simulink model "cpp_m1hp_demo"  (R2022b)
settings: Solver=FixedStepDiscrete  StartTime=0.0  StopTime=6  FixedStep=FEM_Ts  MaxStep=FEM_Ts  RelTol=1e-2
InitFcn:
  | %
  | % Initialization callback function
  | %
  | 
  | try
  |    fprintf('\nGMT IMS version (%s)!\n',simulink_fname );
  | 
  |    % Get Simulink model directory
  |    [filepath,name,ext] = fileparts(which(bdroot));
  | 
  |    if ~strcmp(filepath,pwd)
  |       fprintf('\nChanging current directory to \n %s \n',filepath);
  |       cd(filepath);
  |    end
  | 
  |    %
  |  if(osim.bpless_wl)
  |     fprintf('Generating bumpless wind load time series\n');
  |  end
  | catch
  |    warning('Running the InitFcn from puSimulate script');
  | end
values from neighbouring files (symbols this model uses):
  a_max = 250e-6    (= 0.00025)    [load_im_with_m1act_damp.m]    (also in load_m1hp_cpp_demo.m)
  b = B(:,in)*m1sys{seg}.Kbal    [evalM1ofl_act_damp.m]
  c = [Upsilon*C(out0,:);     C(out1a,:)-C(out1b,:);     C(out2,:)]    [evalM1ofl_act_damp.m]
  delta_sim = 1e-3    (= 0.001)    [load_im_with_m1act_damp.m]    (also in load_m1hp_cpp_demo.m)
  drv_delay = ceil(mount.delay/FEM_Ts)    [load_im_with_m1act_damp.m]    (also in load_m1hp_cpp_demo.m)
  FEM_Ts = 1/1e3    (= 0.001)    [load_im_with_m1act_damp.m]    (also in load_m1hp_cpp_demo.m)
  Hdrive_d = c2d(o.Hdrive(1,1), FEM_Ts, 'tustin')    [load_im_with_m1act_damp.m]    (also in load_m1hp_cpp_demo.m)
  m1sys = ovr_ofl_crtl(m1sys,seg)    [evalM1ofl_act_damp.m]    (also in load_im_with_m1act_damp.m = ovr_ofl_crtl(m1sys))
  o = fun_confBase(oTest)    [load_im_with_m1act_damp.m]    (also in load_m1hp_cpp_demo.m)
  PG = zeros(length(om2),6)    [load_im_with_m1act_damp.m]    (also in load_m1hp_cpp_demo.m)
  phiB = inputs2ModalF(mode_ind_vec,indDesInputs)    [load_im_with_m1act_damp.m]    (also in load_m1hp_cpp_demo.m)
  phiC = modalDisp2Outputs(indDesOutputs,mode_ind_vec)    [load_im_with_m1act_damp.m]    (also in load_m1hp_cpp_demo.m)
  Psi_ss = gainMatrix(indDesOutputs,indDesInputs) - K_ss    [load_im_with_m1act_damp.m]    (also in load_m1hp_cpp_demo.m)
  t_gd = 0*0.5    (= 0)    [load_im_with_m1act_damp.m]    (also in load_m1hp_cpp_demo.m)
  t_gd_v = 0*t_gd    (= 0)    [load_im_with_m1act_damp.m]    (also in load_m1hp_cpp_demo.m)
  Tcmd = 12    [load_im_with_m1act_damp.m]    (also in load_m1hp_cpp_demo.m)
  v0 = 0    [load_im_with_m1act_damp.m]    (also in load_m1hp_cpp_demo.m)
  v_max = 50e-6    (= 5e-05)    [load_im_with_m1act_damp.m]    (also in load_m1hp_cpp_demo.m)
  x0 = 0    [load_im_with_m1act_damp.m]    (also in load_m1hp_cpp_demo.m)
  x0_f = xf(end,:)    [load_im_with_m1act_damp.m]    (also in load_m1hp_cpp_demo.m)
undefined symbols (not defined in the file or in its folder): a, A_f, az, az_ff_en, B_f, C_f, D_f, DiscIntNeverNeededParam, el, gir, magnitude, mount, osim
libraries: simulink x8, ims_block_library x7, simulink_extras x2
(part 1 of 3)
settings Model: PauseTimes=0  Creator=RRomano  LastModifiedBy=rromano
settings SolverCC: MaxConsecutiveMinStep=10  ZeroCrossAlgorithm=Adaptive  AlgebraicLoopSolver=TrustRegion
settings DataIOCC: SaveOutput=off  SignalLogging=off  DSMLogging=off  SaveTime=off  ReturnWorkspaceOutputs=off
settings OptimizationCC: DefaultParameterBehavior=Inlined  StrengthReduction=on  PassReuseOutputArgsAs=Individual arguments  EfficientMapNaN2IntZero=off  SimCompilerOptimization=on  AccelVerboseBuild=on  OptimizeBlockOrder=speed  OptimizationPriority=Speed  OptimizationCustomize=off  MultiThreadedLoops=on  EfficientTunableParamExpr=on
settings DebuggingCC: InheritedTsInSrcMsg=none  MultiTaskRateTransMsg=warning  ParameterTunabilityLossMsg=error  UnconnectedInputMsg=warning  UnconnectedOutputMsg=warning  UnconnectedLineMsg=warning  SFUnexpectedBacktrackingDiag=warning  SFNoUnconditionalDefaultTransitionDiag=warning  SFExecutionAtInitializationDiag=none  SFMachineParentedDataDiag=warning  ArithmeticOperatorsInVariantConditions=warning
settings HardwareCC: ProdBitPerLong=64  ProdHWDeviceType=Intel->x86-64 (Linux 64)  TargetBitPerLong=64  TargetBitPerPointer=64  TargetBitPerSizeT=64  TargetBitPerPtrDiffT=64  TargetLongLongMode=on  TargetIntDivRoundTo=Zero  TargetEndianess=LittleEndian  TargetWordSize=64  TargetHWDeviceType=MATLAB Host  ProdEqTarget=off
settings ModelReferenceCC: EnableRefExpFcnMdlSchedulingChecks=on
settings SFSimCC: SimUseLocalCustomCode=off  MATLABDynamicMemAlloc=off  CustomCodeUndefinedFunction=UseInterfaceOnly
settings RTWCC: Description=Embedded Coder  SystemTargetFile=ert.tlc  GenCodeOnly=on  TemplateMakefile=ert_default_tmf  GenerateReport=on  BuildConfiguration=Faster Runs  IncludeHyperlinkInReport=on  GenerateTraceInfo=on  GenerateTraceReport=on  GenerateTraceReportSl=on  GenerateTraceReportSf=on  GenerateTraceReportEml=on  DLArmComputeVersion=19.05
settings CodeAppCC: ForceParamTrailComments=on  IgnoreCustomStorageClasses=off  MaxIdLength=128  OperatorAnnotations=on  SimulinkDataObjDesc=on  SFDataObjDesc=on  InsertBlockDesc=on  MATLABSourceComments=on
settings ERTTargetCC: GenerateSampleERTMain=on  InlinedParameterPlacement=NonHierarchical  ERTCustomFileTemplate=example_file_process.tlc
settings ConfigComp: CovMetricSettings=dw  CovSaveCumulativeToWorkspaceVar=on  CovSaveSingleToWorkspaceVar=on  CovExternalEMLEnable=off

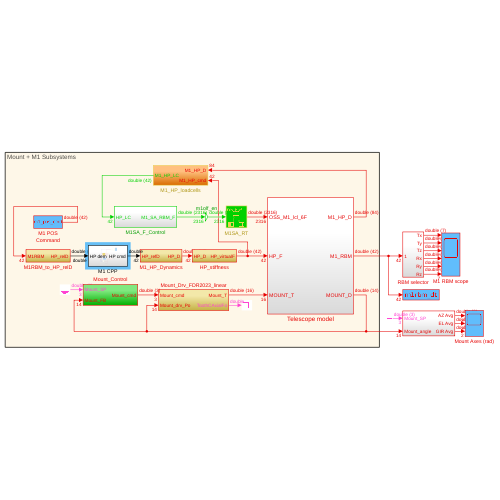
[thumbnail: Simulink's stored preview of the top-level diagram]
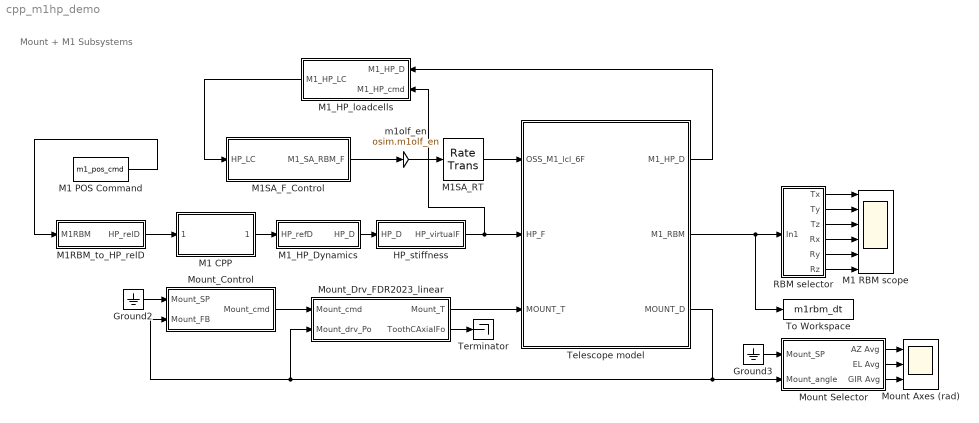
== system cpp_m1hp_demo ==
  note: Mount + M1 Subsystems
  Ground2 : Ground
  Ground3 : Ground
  HP_stiffness : Subsystem
  M1 CPP : Subsystem
  M1 POS Command : FromWorkspace  VariableName=m1_pos_cmd  SampleTime=-1  Interpolate=off  OutputAfterFinalValue=Holding final value
  M1 RBM scope : Scope  NumInputPorts=6
  M1RBM_to_HP_relD : Subsystem
  M1SA_F_Control : Subsystem
  M1SA_RT : RateTransition  Deterministic=off  OutPortSampleTime=FEM_Ts
  M1_HP_Dynamics : Subsystem
  M1_HP_loadcells : Subsystem
  Mount Axes (rad) : Scope  NumInputPorts=3
  Mount Selector : Subsystem
  Mount_Control : Subsystem
  Mount_Drv_FDR2023_linear : Subsystem
  RBM selector : Subsystem
  Telescope model : Subsystem
  Terminator : Terminator
  To Workspace : ToWorkspace  VariableName=m1rbm_dt  SampleTime=-1
  m1olf_en : Gain  Gain=osim.m1olf_en
  wires:
  M1_HP_Dynamics/1(HP_D) -> HP_stiffness/1(HP_D)
  M1SA_F_Control/1(M1_SA_RBM_F) -> m1olf_en/1
  Ground2/1 -> Mount_Control/1(Mount_SP)
  M1_HP_loadcells/1(M1_HP_LC) -> M1SA_F_Control/1(HP_LC)
  Telescope model/3(MOUNT_D) -> Mount Selector/2(Mount_angle), Mount_Drv_FDR2023_linear/2(Mount_drv_Po), Mount_Control/2(Mount_FB)
  Mount_Drv_FDR2023_linear/2(ToothCAxialFo) -> Terminator/1
  Telescope model/1(M1_HP_D) -> M1_HP_loadcells/1(M1_HP_D)
  Mount_Control/1(Mount_cmd) -> Mount_Drv_FDR2023_linear/1(Mount_cmd)
  Mount_Drv_FDR2023_linear/1(Mount_T) -> Telescope model/3(MOUNT_T)
  HP_stiffness/1(HP_virtualF) -> M1_HP_loadcells/2(M1_HP_cmd), Telescope model/2(HP_F)
  RBM selector/1(Tx) -> M1 RBM scope/1
  RBM selector/2(Ty) -> M1 RBM scope/2
  RBM selector/3(Tz) -> M1 RBM scope/3
  RBM selector/4(Rx) -> M1 RBM scope/4
  RBM selector/5(Ry) -> M1 RBM scope/5
  RBM selector/6(Rz) -> M1 RBM scope/6
  Telescope model/2(M1_RBM) -> To Workspace/1, RBM selector/1(In1)
  M1 POS Command/1 -> M1RBM_to_HP_relD/1(M1RBM)
  Mount Selector/1(AZ Avg) -> Mount Axes (rad)/1
  Mount Selector/2(EL Avg) -> Mount Axes (rad)/2
  Mount Selector/3(GIR Avg) -> Mount Axes (rad)/3
  Ground3/1 -> Mount Selector/1(Mount_SP)
  M1SA_RT/1 -> Telescope model/1(OSS_M1_lcl_6F)
  m1olf_en/1 -> M1SA_RT/1
  M1RBM_to_HP_relD/1(HP_relD) -> M1 CPP/1(HP dem)
  M1 CPP/1(HP cmd) -> M1_HP_Dynamics/1(HP_refD)

== system cpp_m1hp_demo/HP_stiffness ==
  note: This block takes HP reference relative displacements (lengths) and provides the virtual forces to enforce such a displacement. The force output also corrects (offsets) the HP load cell measurement by the commanded change in position.
  note: Offset displacement, used in calculation of hard point forces.
  note: The virtual force simulates the extension
      | of the HP by applying and equal and
      | opposite force on the face of the mirror and cell.
  note: HP virtual
      | forces (N)
  HP_D : Inport
  Demux1 : Demux  Outputs=6*ones(7,1)
  HpK1 : Gain  Gain=m1sys{2}.HPstiff
  HpK2 : Gain  Gain=m1sys{3}.HPstiff
  HpK3 : Gain  Gain=m1sys{5}.HPstiff
  HpK4 : Gain  Gain=m1sys{6}.HPstiff
  HpK5 : Gain  Gain=m1sys{4}.HPstiff
  HpK6 : Gain  Gain=m1sys{7}.HPstiff
  HpK8 : Gain  Gain=m1sys{1}.HPstiff
  Mux3 : Mux  Inputs=6*ones(7,1)
  HP_virtualF : Outport  VectorParamsAs1DForOutWhenUnconnected=off
  wires:
  Mux3/1 -> HP_virtualF/1
  HpK8/1 -> Mux3/1
  HpK6/1 -> Mux3/7
  HpK1/1 -> Mux3/2
  HpK2/1 -> Mux3/3
  HpK5/1 -> Mux3/4
  HpK3/1 -> Mux3/5
  HpK4/1 -> Mux3/6
  Demux1/1 -> HpK8/1
  HP_D/1 -> Demux1/1
  Demux1/2 -> HpK1/1
  Demux1/3 -> HpK2/1
  Demux1/4 -> HpK5/1
  Demux1/5 -> HpK3/1
  Demux1/6 -> HpK4/1
  Demux1/7 -> HpK6/1

== system cpp_m1hp_demo/M1 CPP ==
  HP dem : Inport
  Constant : Constant  Value=osim.m1cpp_en  VectorParams1D=off
  Ground1 : Ground
  HP scope : Scope  NumInputPorts=6
  HP selector : Subsystem
  M1CPP_RT : RateTransition  Integrity=off  Deterministic=off  OutPortSampleTime=Tcmd
  M1CPP_RT1 : RateTransition  Integrity=off  Deterministic=off
  Mux2 : Mux  Inputs=2
  Mux3 : Mux  Inputs=2
  Selector : Selector  InputPortWidth=42  IndexOptions=Index vector (dialog)  Indices=[7:42]  OutputSizes=1
  Selector1 : Selector  InputPortWidth=42  IndexOptions=Index vector (dialog)  Indices=[1:6]  OutputSizes=1
  Switch : Switch  Criteria=u2 ~= 0  SaturateOnIntegerOverflow=off  InputSameDT=off
  Terminator1 : Terminator
  Terminator2 : Terminator
  cmd_pre_proc : Subsystem
  HP cmd : Outport
  wires:
  HP selector/3(HP3) -> HP scope/3
  HP selector/2(HP2) -> HP scope/2
  HP selector/1(HP1) -> HP scope/1
  cmd_pre_proc/2(vel_d) -> Terminator1/1
  Switch/1 -> HP cmd/1
  HP selector/5(HP5) -> HP scope/5
  Mux3/1 -> M1CPP_RT1/1
  HP selector/6(HP6) -> HP scope/6
  HP selector/4(HP4) -> HP scope/4
  HP dem/1 -> Switch/3, M1CPP_RT/1
  cmd_pre_proc/3(acc_d) -> Terminator2/1
  M1CPP_RT1/1 -> Switch/1
  Selector/1 -> Mux3/2
  Selector1/1 -> cmd_pre_proc/1(x_target), Mux2/1
  Ground1/1 -> cmd_pre_proc/2(v_target)
  Constant/1 -> Switch/2
  M1CPP_RT/1 -> Selector/1, Selector1/1
  Mux2/1 -> HP selector/1(In1)
  cmd_pre_proc/1(pos_d) -> Mux2/2, Mux3/1

== system cpp_m1hp_demo/M1RBM_to_HP_relD ==
  note: CG desired
      | displacement/rotation
  note: This block converts from CG displacements and rotations,
      | and converts to Hard Point lengths.  Hard point lengths are
      | changed by applying an equal and opposite force to the hard
      | point, and then offseting output by the commanded change
      | in position.
  note: Hexapod Desired
      | Displacements
  note: Offset displacement, used in calculation of hard point forces.
  M1RBM : Inport
  CG2HpS1 : Gain  Gain=m1sys{1}.M1RBM2HP  Multiplication=Matrix(K*u)
  CG2HpS2 : Gain  Gain=m1sys{2}.M1RBM2HP  Multiplication=Matrix(K*u)
  CG2HpS3 : Gain  Gain=m1sys{3}.M1RBM2HP  Multiplication=Matrix(K*u)
  CG2HpS4 : Gain  Gain=m1sys{4}.M1RBM2HP  Multiplication=Matrix(K*u)
  CG2HpS5 : Gain  Gain=m1sys{5}.M1RBM2HP  Multiplication=Matrix(K*u)
  CG2HpS6 : Gain  Gain=m1sys{6}.M1RBM2HP  Multiplication=Matrix(K*u)
  CG2HpS7 : Gain  Gain=m1sys{7}.M1RBM2HP  Multiplication=Matrix(K*u)
  Demux1 : Demux  Outputs=6*ones(7,1)
  Mux3 : Mux  Inputs=6*ones(7,1)
  HP_relD : Outport  VectorParamsAs1DForOutWhenUnconnected=off
  wires:
  Mux3/1 -> HP_relD/1
  Demux1/2 -> CG2HpS2/1
  Demux1/3 -> CG2HpS3/1
  Demux1/4 -> CG2HpS4/1
  Demux1/5 -> CG2HpS5/1
  Demux1/6 -> CG2HpS6/1
  Demux1/1 -> CG2HpS1/1
  Demux1/7 -> CG2HpS7/1
  CG2HpS1/1 -> Mux3/1
  M1RBM/1 -> Demux1/1
  CG2HpS2/1 -> Mux3/2
  CG2HpS3/1 -> Mux3/3
  CG2HpS4/1 -> Mux3/4
  CG2HpS5/1 -> Mux3/5
  CG2HpS6/1 -> Mux3/6
  CG2HpS7/1 -> Mux3/7

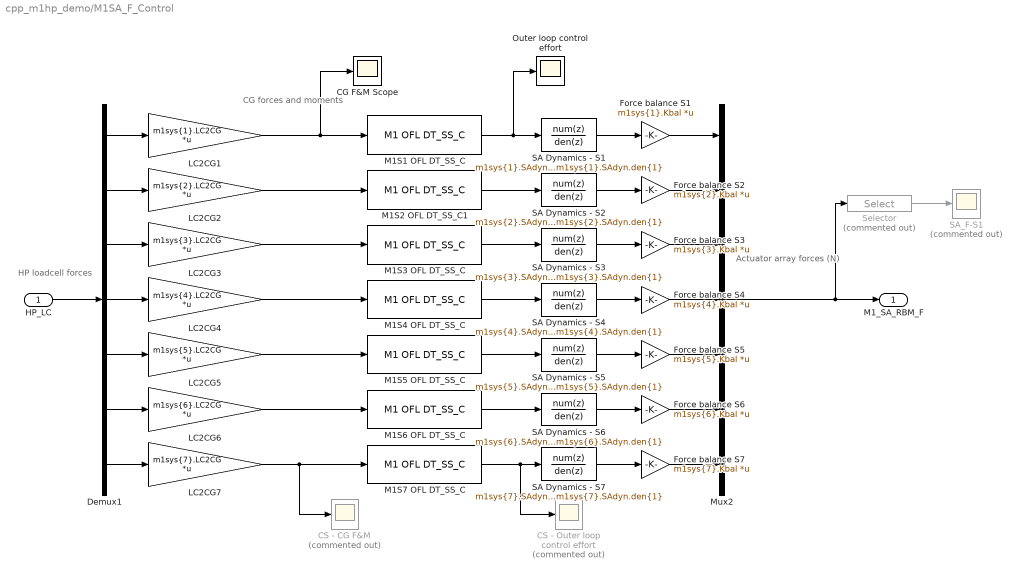
== system cpp_m1hp_demo/M1SA_F_Control ==
  note: HP loadcell forces
  note: Actuator array
      | forces (N)
  note: CG forces
      | and moments
  HP_LC : Inport
  CG F&M Scope : Scope
  CS - CG F&M : Scope  Commented=on
  CS - Outer loop control effort : Scope  Commented=on
  Demux1 : Demux  Outputs=6*ones(7,1)
  Force balance S1 : Gain  Gain=m1sys{1}.Kbal  Multiplication=Matrix(K*u)
  Force balance S2 : Gain  Gain=m1sys{2}.Kbal  Multiplication=Matrix(K*u)
  Force balance S3 : Gain  Gain=m1sys{3}.Kbal  Multiplication=Matrix(K*u)
  Force balance S4 : Gain  Gain=m1sys{4}.Kbal  Multiplication=Matrix(K*u)
  Force balance S5 : Gain  Gain=m1sys{5}.Kbal  Multiplication=Matrix(K*u)
  Force balance S6 : Gain  Gain=m1sys{6}.Kbal  Multiplication=Matrix(K*u)
  Force balance S7 : Gain  Gain=m1sys{7}.Kbal  Multiplication=Matrix(K*u)
  LC2CG1 : Gain  Gain=m1sys{1}.LC2CG  Multiplication=Matrix(K*u)
  LC2CG2 : Gain  Gain=m1sys{2}.LC2CG  Multiplication=Matrix(K*u)
  LC2CG3 : Gain  Gain=m1sys{3}.LC2CG  Multiplication=Matrix(K*u)
  LC2CG4 : Gain  Gain=m1sys{4}.LC2CG  Multiplication=Matrix(K*u)
  LC2CG5 : Gain  Gain=m1sys{5}.LC2CG  Multiplication=Matrix(K*u)
  LC2CG6 : Gain  Gain=m1sys{6}.LC2CG  Multiplication=Matrix(K*u)
  LC2CG7 : Gain  Gain=m1sys{7}.LC2CG  Multiplication=Matrix(K*u)
  M1S1 OFL DT_SS_C : ims_block_library/M1 OFL DT_SS_C  dt_SS_struct=m1sys{1}.ofl.SSdtC
  M1S2 OFL DT_SS_C1 : ims_block_library/M1 OFL DT_SS_C  dt_SS_struct=m1sys{2}.ofl.SSdtC
  M1S3 OFL DT_SS_C : ims_block_library/M1 OFL DT_SS_C  dt_SS_struct=m1sys{3}.ofl.SSdtC
  M1S4 OFL DT_SS_C : ims_block_library/M1 OFL DT_SS_C  dt_SS_struct=m1sys{4}.ofl.SSdtC
  M1S5 OFL DT_SS_C : ims_block_library/M1 OFL DT_SS_C  dt_SS_struct=m1sys{5}.ofl.SSdtC
  M1S6 OFL DT_SS_C : ims_block_library/M1 OFL DT_SS_C  dt_SS_struct=m1sys{6}.ofl.SSdtC
  M1S7 OFL DT_SS_C : ims_block_library/M1 OFL DT_SS_C  dt_SS_struct=m1sys{7}.ofl.SSdtC
  Mux2 : Mux  Inputs=7
  Outer loop control effort : Scope
  SA Dynamics - S1 : DiscreteTransferFcn  Numerator=m1sys{1}.SAdyn.num{1}  Denominator=m1sys{1}.SAdyn.den{1}  SampleTime=m1sys{1}.ofl.Ts  a0EqualsOne=on
  SA Dynamics - S2 : DiscreteTransferFcn  Numerator=m1sys{2}.SAdyn.num{1}  Denominator=m1sys{2}.SAdyn.den{1}  SampleTime=m1sys{1}.ofl.SSdtC{1}.Ts  a0EqualsOne=on
  SA Dynamics - S3 : DiscreteTransferFcn  Numerator=m1sys{3}.SAdyn.num{1}  Denominator=m1sys{3}.SAdyn.den{1}  SampleTime=m1sys{1}.ofl.SSdtC{1}.Ts  a0EqualsOne=on
  SA Dynamics - S4 : DiscreteTransferFcn  Numerator=m1sys{4}.SAdyn.num{1}  Denominator=m1sys{4}.SAdyn.den{1}  SampleTime=m1sys{1}.ofl.SSdtC{1}.Ts  a0EqualsOne=on
  SA Dynamics - S5 : DiscreteTransferFcn  Numerator=m1sys{5}.SAdyn.num{1}  Denominator=m1sys{5}.SAdyn.den{1}  SampleTime=m1sys{1}.ofl.SSdtC{1}.Ts  a0EqualsOne=on
  SA Dynamics - S6 : DiscreteTransferFcn  Numerator=m1sys{6}.SAdyn.num{1}  Denominator=m1sys{6}.SAdyn.den{1}  SampleTime=m1sys{1}.ofl.SSdtC{1}.Ts  a0EqualsOne=on
  SA Dynamics - S7 : DiscreteTransferFcn  Numerator=m1sys{7}.SAdyn.num{1}  Denominator=m1sys{7}.SAdyn.den{1}  SampleTime=m1sys{1}.ofl.SSdtC{1}.Ts  a0EqualsOne=on
  SA_F-S1 : Scope  Commented=on
  Selector : Selector  Commented=on  InputPortWidth=2316  IndexOptions=Index vector (dialog)  Indices=[1:335]  OutputSizes=1
  M1_SA_RBM_F : Outport  VectorParamsAs1DForOutWhenUnconnected=off
  wires:
  HP_LC/1 -> Demux1/1
  M1S1 OFL DT_SS_C/1 -> Outer loop control effort/1, SA Dynamics - S1/1
  M1S2 OFL DT_SS_C1/1 -> SA Dynamics - S2/1
  M1S3 OFL DT_SS_C/1 -> SA Dynamics - S3/1
  M1S4 OFL DT_SS_C/1 -> SA Dynamics - S4/1
  M1S5 OFL DT_SS_C/1 -> SA Dynamics - S5/1
  M1S6 OFL DT_SS_C/1 -> SA Dynamics - S6/1
  M1S7 OFL DT_SS_C/1 -> CS - Outer loop control effort/1, SA Dynamics - S7/1
  LC2CG7/1 -> M1S7 OFL DT_SS_C/1, CS - CG F&M/1
  LC2CG6/1 -> M1S6 OFL DT_SS_C/1
  LC2CG5/1 -> M1S5 OFL DT_SS_C/1
  LC2CG4/1 -> M1S4 OFL DT_SS_C/1
  LC2CG3/1 -> M1S3 OFL DT_SS_C/1
  LC2CG2/1 -> M1S2 OFL DT_SS_C1/1
  LC2CG1/1 -> M1S1 OFL DT_SS_C/1, CG F&M Scope/1
  Demux1/1 -> LC2CG1/1
  Demux1/2 -> LC2CG2/1
  Demux1/3 -> LC2CG3/1
  Demux1/4 -> LC2CG4/1
  Demux1/5 -> LC2CG5/1
  Demux1/6 -> LC2CG6/1
  Demux1/7 -> LC2CG7/1
  Force balance S2/1 -> Mux2/2
  Force balance S3/1 -> Mux2/3
  Force balance S4/1 -> Mux2/4
  Force balance S6/1 -> Mux2/6
  Force balance S5/1 -> Mux2/5
  Force balance S7/1 -> Mux2/7
  Mux2/1 -> M1_SA_RBM_F/1, Selector/1
  SA Dynamics - S1/1 -> Force balance S1/1
  SA Dynamics - S2/1 -> Force balance S2/1
  SA Dynamics - S3/1 -> Force balance S3/1
  SA Dynamics - S4/1 -> Force balance S4/1
  SA Dynamics - S5/1 -> Force balance S5/1
  SA Dynamics - S6/1 -> Force balance S6/1
  SA Dynamics - S7/1 -> Force balance S7/1
  Selector/1 -> SA_F-S1/1
  Force balance S1/1 -> Mux2/1

== system cpp_m1hp_demo/M1_HP_Dynamics ==
  note: This block takes HP reference relative displacements (lengths) and provides its relative displacements subject to a linear dyamics.
  note: Hexapod Desired
      | Displacements
  note: HP Offset displacement, used in calculation of hard point forces.
  note: HP displacement closed-loop dynamics
  HP_refD : Inport
  Demux1 : Demux  Outputs=6*ones(7,1)
  Mux3 : Mux  Inputs=6*ones(7,1)
  S1HP_dyn_dTF : DiscreteTransferFcn  Numerator=m1sys{1}.HPdtf.num{1}  Denominator=m1sys{1}.HPdtf.den{1}  SampleTime=m1sys{1}.HPdtf.Ts  a0EqualsOne=on
  S2HP_dyn_dTF : DiscreteTransferFcn  Numerator=m1sys{2}.HPdtf.num{1}  Denominator=m1sys{2}.HPdtf.den{1}  SampleTime=m1sys{2}.HPdtf.Ts  a0EqualsOne=on
  S3HP_dyn_dTF : DiscreteTransferFcn  Numerator=m1sys{3}.HPdtf.num{1}  Denominator=m1sys{3}.HPdtf.den{1}  SampleTime=m1sys{3}.HPdtf.Ts  a0EqualsOne=on
  S4HP_dyn_dTF : DiscreteTransferFcn  Numerator=m1sys{4}.HPdtf.num{1}  Denominator=m1sys{4}.HPdtf.den{1}  SampleTime=m1sys{4}.HPdtf.Ts  a0EqualsOne=on
  S5HP_dyn_dTF : DiscreteTransferFcn  Numerator=m1sys{5}.HPdtf.num{1}  Denominator=m1sys{5}.HPdtf.den{1}  SampleTime=m1sys{5}.HPdtf.Ts  a0EqualsOne=on
  S6HP_dyn_dTF : DiscreteTransferFcn  Numerator=m1sys{6}.HPdtf.num{1}  Denominator=m1sys{6}.HPdtf.den{1}  SampleTime=m1sys{6}.HPdtf.Ts  a0EqualsOne=on
  S7HP_dyn_dTF : DiscreteTransferFcn  Numerator=m1sys{7}.HPdtf.num{1}  Denominator=m1sys{7}.HPdtf.den{1}  SampleTime=m1sys{7}.HPdtf.Ts  a0EqualsOne=on
  HP_D : Outport  VectorParamsAs1DForOutWhenUnconnected=off
  wires:
  Mux3/1 -> HP_D/1
  Demux1/1 -> S1HP_dyn_dTF/1
  HP_refD/1 -> Demux1/1
  Demux1/2 -> S2HP_dyn_dTF/1
  Demux1/3 -> S3HP_dyn_dTF/1
  Demux1/4 -> S4HP_dyn_dTF/1
  Demux1/5 -> S5HP_dyn_dTF/1
  Demux1/6 -> S6HP_dyn_dTF/1
  Demux1/7 -> S7HP_dyn_dTF/1
  S1HP_dyn_dTF/1 -> Mux3/1
  S2HP_dyn_dTF/1 -> Mux3/2
  S3HP_dyn_dTF/1 -> Mux3/3
  S4HP_dyn_dTF/1 -> Mux3/4
  S5HP_dyn_dTF/1 -> Mux3/5
  S6HP_dyn_dTF/1 -> Mux3/6
  S7HP_dyn_dTF/1 -> Mux3/7

== system cpp_m1hp_demo/M1_HP_loadcells ==
  note: This block converts from CG displacements and rotations,
      | and converts to Hard Point lengths.  Hard point lengths are
      | changed by applying an equal and opposite force to the hard
      | point, and then offseting output by the commanded change
      | in position.
  note: Hexapod Offset Forces
  note: LC Forces (N)
  M1_HP_D : Inport
  M1_HP_cmd : Inport  Port=2
  Demux1 : Demux  Outputs=6*ones(7,1)
  Demux2 : Demux  Outputs=6*ones(14,1);%6*ones(7,1)
  M1S1 Loadcell : Subsystem
  M1S2 Loadcell : Subsystem
  M1S3 Loadcell : Subsystem
  M1S4 Loadcell : Subsystem
  M1S5 Loadcell : Subsystem
  M1S6 Loadcell : Subsystem
  M1S7 Control : Subsystem
  Mux2 : Mux  Inputs=7
  Rate Transition1 : RateTransition  Integrity=off  Deterministic=off  OutPortSampleTime=m1sys{1}.ofl.SSdtC{1}.Ts
  Rate Transition2 : RateTransition  Integrity=off  Deterministic=off  OutPortSampleTime=m1sys{1}.ofl.SSdtC{1}.Ts
  M1_HP_LC : Outport  VectorParamsAs1DForOutWhenUnconnected=off
  wires:
  Demux2/9 -> M1S5 Loadcell/2(HP_D_cell)
  Demux2/3 -> M1S2 Loadcell/2(HP_D_cell)
  Demux2/5 -> M1S3 Loadcell/2(HP_D_cell)
  Demux2/13 -> M1S7 Control/2(HP_D_cell)
  Demux2/11 -> M1S6 Loadcell/2(HP_D_cell)
  Demux2/4 -> M1S2 Loadcell/3(HP_D_face)
  Demux2/6 -> M1S3 Loadcell/3(HP_D_face)
  Demux2/10 -> M1S5 Loadcell/3(HP_D_face)
  Demux2/12 -> M1S6 Loadcell/3(HP_D_face)
  Demux2/14 -> M1S7 Control/3(HP_D_face)
  M1_HP_D/1 -> Rate Transition1/1
  M1S1 Loadcell/1(HP_F_meas) -> Mux2/1
  M1S2 Loadcell/1(HP_F_meas) -> Mux2/2
  M1S3 Loadcell/1(HP_F_meas) -> Mux2/3
  M1S5 Loadcell/1(HP_F_meas) -> Mux2/5
  M1S6 Loadcell/1(HP_F_meas) -> Mux2/6
  M1S7 Control/1(HP_F_meas) -> Mux2/7
  Demux2/2 -> M1S1 Loadcell/3(HP_D_face)
  Demux2/1 -> M1S1 Loadcell/2(HP_D_cell)
  M1S4 Loadcell/1(HP_F_meas) -> Mux2/4
  Demux2/7 -> M1S4 Loadcell/2(HP_D_cell)
  Demux2/8 -> M1S4 Loadcell/3(HP_D_face)
  M1_HP_cmd/1 -> Rate Transition2/1
  Demux1/1 -> M1S1 Loadcell/1(HP_F_cmd)
  Demux1/2 -> M1S2 Loadcell/1(HP_F_cmd)
  Demux1/3 -> M1S3 Loadcell/1(HP_F_cmd)
  Demux1/4 -> M1S4 Loadcell/1(HP_F_cmd)
  Demux1/5 -> M1S5 Loadcell/1(HP_F_cmd)
  Demux1/6 -> M1S6 Loadcell/1(HP_F_cmd)
  Demux1/7 -> M1S7 Control/1(HP_F_cmd)
  Mux2/1 -> M1_HP_LC/1
  Rate Transition2/1 -> Demux1/1
  Rate Transition1/1 -> Demux2/1

== system cpp_m1hp_demo/Mount Selector ==
  note: Motion in rad
  Mount_SP : Inport
  Mount_angle : Inport  Port=2
  Demux1 : Demux  Outputs=[1,1,1]
  Demux3 : Demux  Outputs=3
  Drv_Pos_avg : Gain  Gain=blkdiag(1/4*ones(1,4),1/6*ones(1,6),1/4*ones(1,4))  Multiplication=Matrix(K*u) (u vector)
  Mux : Mux  Inputs=2
  Mux1 : Mux  Inputs=2
  Mux2 : Mux  Inputs=2
  To Workspace2 : ToWorkspace  VariableName=mnt_dt  SampleTime=-1
  AZ Avg : Outport  VectorParamsAs1DForOutWhenUnconnected=off
  EL Avg : Outport  Port=2  VectorParamsAs1DForOutWhenUnconnected=off
  GIR Avg : Outport  Port=3  VectorParamsAs1DForOutWhenUnconnected=off
  wires:
  Mount_angle/1 -> Drv_Pos_avg/1
  Mux/1 -> AZ Avg/1
  Demux3/1 -> Mux/2
  Mux1/1 -> EL Avg/1
  Demux3/2 -> Mux1/2
  Demux3/3 -> Mux2/2
  Mux2/1 -> GIR Avg/1
  Mount_SP/1 -> Demux1/1
  Demux1/3 -> Mux2/1
  Demux1/1 -> Mux/1
  Demux1/2 -> Mux1/1
  Drv_Pos_avg/1 -> To Workspace2/1, Demux3/1

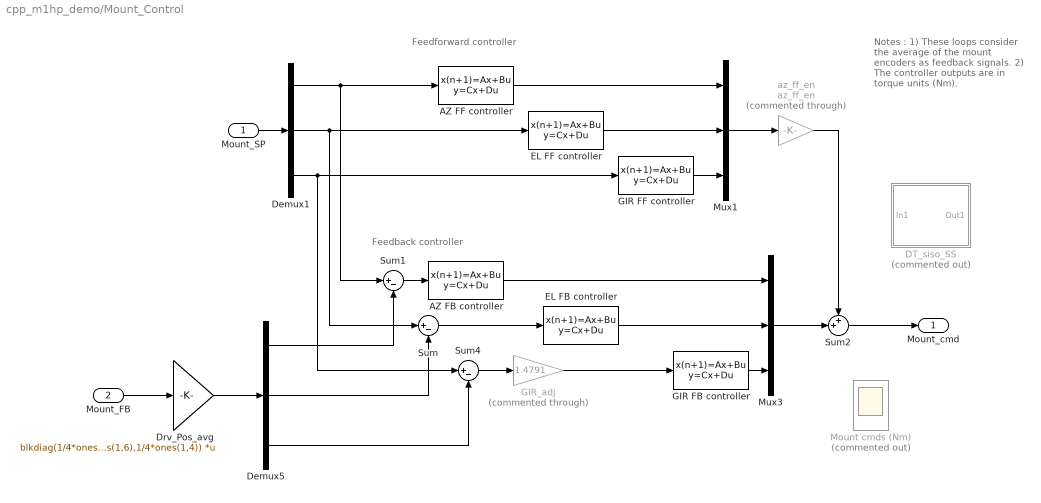
== system cpp_m1hp_demo/Mount_Control ==
  note: Feedback controller
  note: Feedforward controller
  note: Notes :
      | 1) These loops consider the average of the mount encoders as feedback signals.
      | 2) The controller outputs are in torque units (Nm).
  Mount_SP : Inport
  Mount_FB : Inport  Port=2
  AZ FB controller : DiscreteStateSpace  A=mount.az.SSdtHfb.A  B=mount.az.SSdtHfb.B  C=mount.az.SSdtHfb.C  D=mount.az.SSdtHfb.D  SampleTime=mount.az.SSdtHfb.Ts
  AZ FF controller : DiscreteStateSpace  A=mount.az.SSdtHff.A  B=mount.az.SSdtHff.B  C=mount.az.SSdtHff.C  D=mount.az.SSdtHff.D  SampleTime=mount.az.SSdtHff.Ts
  DT_siso_SS : Subsystem  Commented=on
  Demux1 : Demux  Outputs=[1,1,1]
  Demux5 : Demux  Outputs=3
  Drv_Pos_avg : Gain  Gain=blkdiag(1/4*ones(1,4),1/6*ones(1,6),1/4*ones(1,4))  Multiplication=Matrix(K*u) (u vector)
  EL FB controller : DiscreteStateSpace  A=mount.el.SSdtHfb.A  B=mount.el.SSdtHfb.B  C=mount.el.SSdtHfb.C  D=mount.el.SSdtHfb.D  SampleTime=mount.el.SSdtHfb.Ts
  EL FF controller : DiscreteStateSpace  A=mount.el.SSdtHff.A  B=mount.el.SSdtHff.B  C=mount.el.SSdtHff.C  D=mount.el.SSdtHff.D  SampleTime=mount.el.SSdtHff.Ts
  GIR FB controller : DiscreteStateSpace  A=mount.gir.SSdtHfb.A  B=mount.gir.SSdtHfb.B  C=mount.gir.SSdtHfb.C  D=mount.gir.SSdtHfb.D  SampleTime=mount.gir.SSdtHfb.Ts
  GIR FF controller : DiscreteStateSpace  A=mount.gir.SSdtHff.A  B=mount.gir.SSdtHff.B  C=mount.gir.SSdtHff.C  D=mount.gir.SSdtHff.D  SampleTime=mount.gir.SSdtHff.Ts
  GIR_adj : Gain  Commented=through  Gain=1.4791
  Mount cmds (Nm) : Scope  Commented=on  NumInputPorts=3
  Mux1 : Mux  Inputs=[1,1,1]
  Mux3 : Mux  Inputs=[1,1,1]
  Sum : Sum  Inputs=|+-
  Sum1 : Sum  Inputs=|+-
  Sum2 : Sum  Inputs=++|
  Sum4 : Sum  Inputs=|+-
  az_ff_en : Gain  Commented=through  Gain=az_ff_en
  Mount_cmd : Outport  VectorParamsAs1DForOutWhenUnconnected=off
  wires:
  Mount_FB/1 -> Drv_Pos_avg/1
  Sum1/1 -> AZ FB controller/1
  Demux1/3 -> Sum4/1, GIR FF controller/1
  Mount_SP/1 -> Demux1/1
  Demux1/2 -> Sum/1, EL FF controller/1
  Sum/1 -> EL FB controller/1
  AZ FF controller/1 -> Mux1/1
  EL FF controller/1 -> Mux1/2
  Mux3/1 -> Sum2/2
  Sum2/1 -> Mount_cmd/1
  GIR FF controller/1 -> Mux1/3
  AZ FB controller/1 -> Mux3/1
  EL FB controller/1 -> Mux3/2
  Mux1/1 -> az_ff_en/1
  Sum4/1 -> GIR_adj/1
  GIR FB controller/1 -> Mux3/3
  Demux5/3 -> Sum4/2
  az_ff_en/1 -> Sum2/1
  Demux1/1 -> Sum1/1, AZ FF controller/1
  Drv_Pos_avg/1 -> Demux5/1
  Demux5/2 -> Sum/2
  Demux5/1 -> Sum1/2
  GIR_adj/1 -> GIR FB controller/1

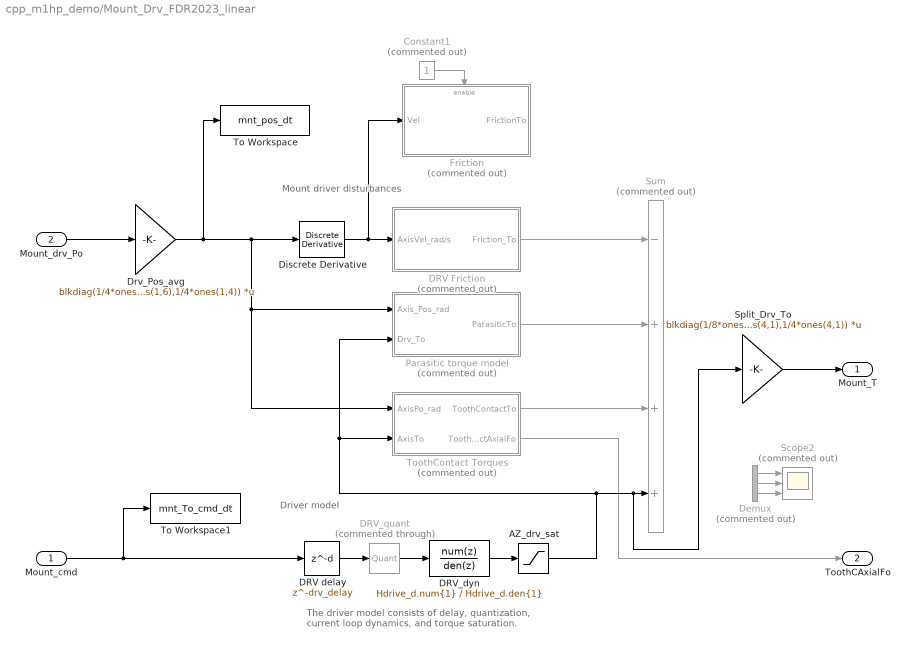
== system cpp_m1hp_demo/Mount_Drv_FDR2023_linear ==
  note: Driver model
  note: The driver model consists of delay, quantization, current loop dynamics, and torque saturation.
  note: Mount driver disturbances
  Mount_cmd : Inport
  Mount_drv_Po : Inport  Port=2
  AZ_drv_sat : Saturate  UpperLimit=o.vTmax  LowerLimit=-o.vTmax
  Constant1 : Constant  Commented=on
  DRV Friction : Subsystem  Commented=on
  DRV delay : Delay  DelayLength=drv_delay  UseCircularBuffer=on  SampleTime=FEM_Ts
  DRV_dyn : DiscreteTransferFcn  Numerator=Hdrive_d.num{1}  Denominator=Hdrive_d.den{1}  SampleTime=FEM_Ts  a0EqualsOne=on
  DRV_quant : Quantizer  Commented=through  QuantizationInterval=o.vMotQuant_Nm
  Demux : Demux  Commented=on  Outputs=3
  Discrete Derivative : simulink/Discrete/Discrete Derivative  gainval=1  ICPrevScaledInput=0.0  OutMin=[]  OutMax=[]  OutDataType=fixdt(1, 16)  OutScaling=2^-10  DoSatur=off
  Drv_Pos_avg : Gain  Gain=blkdiag(1/4*ones(1,4),1/6*ones(1,6),1/4*ones(1,4))  Multiplication=Matrix(K*u) (u vector)
  Friction : Subsystem  Commented=on
  Parasitic torque model : Subsystem  Commented=on
  Scope2 : Scope  Commented=on  NumInputPorts=3
  Split_Drv_To : Gain  Gain=blkdiag(1/8*ones(8,1),1/4*ones(4,1),1/4*ones(4,1))  Multiplication=Matrix(K*u) (u vector)
  Sum : Sum  Commented=on  Inputs=-+++
  To Workspace : ToWorkspace  VariableName=mnt_pos_dt  SaveFormat=Structure With Time  SampleTime=-1
  To Workspace1 : ToWorkspace  VariableName=mnt_To_cmd_dt  SaveFormat=Structure With Time  SampleTime=-1
  ToothContact Torques : Subsystem  Commented=on
  Mount_T : Outport  VectorParamsAs1DForOutWhenUnconnected=off
  ToothCAxialFo : Outport  Port=2  InitialOutput=0
  wires:
  ToothContact Torques/2(ToothContactAxialFo) -> ToothCAxialFo/1
  Mount_drv_Po/1 -> Drv_Pos_avg/1
  Demux/3 -> Scope2/3
  Demux/1 -> Scope2/1
  Demux/2 -> Scope2/2
  DRV delay/1 -> DRV_quant/1
  Mount_cmd/1 -> To Workspace1/1, DRV delay/1
  DRV_quant/1 -> DRV_dyn/1
  DRV_dyn/1 -> AZ_drv_sat/1
  Drv_Pos_avg/1 -> To Workspace/1, Discrete Derivative/1, Parasitic torque model/1(Axis_Pos_rad), ToothContact Torques/1(AxisPo_rad)
  Split_Drv_To/1 -> Mount_T/1
  Constant1/1 -> Friction/Enable
  Discrete Derivative/1 -> Friction/1(Vel), DRV Friction/1(AxisVel_rad/s)
  AZ_drv_sat/1 -> Split_Drv_To/1, Sum/4, Parasitic torque model/2(Drv_To), ToothContact Torques/2(AxisTo)
  DRV Friction/1(Friction_To) -> Sum/1
  Parasitic torque model/1(ParasiticTo) -> Sum/2
  ToothContact Torques/1(ToothContactTo) -> Sum/3

== system cpp_m1hp_demo/RBM selector ==
  note: Local motion of M1 segments (in m and rad)
  In1 : Inport
  Selector : Selector  InputPortWidth=42  IndexOptions=Index vector (dialog)  Indices=[1:6:42]  OutputSizes=1
  Selector1 : Selector  InputPortWidth=42  IndexOptions=Index vector (dialog)  Indices=[2:6:42]  OutputSizes=1
  Selector2 : Selector  InputPortWidth=42  IndexOptions=Index vector (dialog)  Indices=[3:6:42]  OutputSizes=1
  Selector3 : Selector  InputPortWidth=42  IndexOptions=Index vector (dialog)  Indices=[4:6:42]  OutputSizes=1
  Selector4 : Selector  InputPortWidth=42  IndexOptions=Index vector (dialog)  Indices=[5:6:42]  OutputSizes=1
  Selector5 : Selector  InputPortWidth=42  IndexOptions=Index vector (dialog)  Indices=[6:6:42]  OutputSizes=1
  Tx : Outport  VectorParamsAs1DForOutWhenUnconnected=off
  Ty : Outport  Port=2  VectorParamsAs1DForOutWhenUnconnected=off
  Tz : Outport  Port=3  VectorParamsAs1DForOutWhenUnconnected=off
  Rx : Outport  Port=4  VectorParamsAs1DForOutWhenUnconnected=off
  Ry : Outport  Port=5  VectorParamsAs1DForOutWhenUnconnected=off
  Rz : Outport  Port=6  VectorParamsAs1DForOutWhenUnconnected=off
  wires:
  In1/1 -> Selector3/1, Selector4/1, Selector5/1, Selector/1, Selector1/1, Selector2/1
  Selector/1 -> Tx/1
  Selector4/1 -> Ry/1
  Selector1/1 -> Ty/1
  Selector3/1 -> Rx/1
  Selector5/1 -> Rz/1
  Selector2/1 -> Tz/1

== system cpp_m1hp_demo/Telescope model ==
  OSS_M1_lcl_6F : Inport
  HP_F : Inport  Port=2
  MOUNT_T : Inport  Port=3
  Demux1 : Demux  Outputs=[8,4,4]
  Demux2 : Demux  Outputs=[335,335,335,335,335,335,306]
  Ground : Ground
  Mux2 : Mux  Inputs=[4,6,4]
  Structural Dynamics GMT : Subsystem
  M1_HP_D : Outport  VectorParamsAs1DForOutWhenUnconnected=off
  M1_RBM : Outport  Port=2  VectorParamsAs1DForOutWhenUnconnected=off
  MOUNT_D : Outport  Port=3  VectorParamsAs1DForOutWhenUnconnected=off
  wires:
  MOUNT_T/1 -> Demux1/1
  Demux2/1 -> Structural Dynamics GMT/5(M1_actuators_segment_1(335) [5])
  Demux2/2 -> Structural Dynamics GMT/6(M1_actuators_segment_2(335) [6])
  Demux2/3 -> Structural Dynamics GMT/7(M1_actuators_segment_3(335) [7])
  Demux2/4 -> Structural Dynamics GMT/8(M1_actuators_segment_4(335) [8])
  Demux2/5 -> Structural Dynamics GMT/9(M1_actuators_segment_5(335) [9])
  Demux2/6 -> Structural Dynamics GMT/10(M1_actuators_segment_6(335) [10])
  Demux2/7 -> Structural Dynamics GMT/11(M1_actuators_segment_7(306) [11])
  OSS_M1_lcl_6F/1 -> Demux2/1
  Structural Dynamics GMT/5(OSS_M1_lcl(42) [5]) -> M1_RBM/1
  Demux1/1 -> Structural Dynamics GMT/2(OSS_AzDrive_Torque(8) [2])
  Demux1/2 -> Structural Dynamics GMT/1(OSS_ElDrive_Torque(4) [1])
  Demux1/3 -> Structural Dynamics GMT/3(OSS_RotDrive_Torque(4) [3])
  HP_F/1 -> Structural Dynamics GMT/4(OSS_Harpoint_delta_F(42) [4])
  Structural Dynamics GMT/4(OSS_Hardpoint_D(84) [4]) -> M1_HP_D/1
  Structural Dynamics GMT/1(OSS_ElEncoder_Angle(6) [1]) -> Mux2/2
  Mux2/1 -> MOUNT_D/1
  Structural Dynamics GMT/2(OSS_AzEncoder_Angle(4) [2]) -> Mux2/1
  Structural Dynamics GMT/3(OSS_RotEncoder_Angle(4) [3]) -> Mux2/3
  Ground/1 -> Structural Dynamics GMT/12(OSS_M1_lcl_6F(42) [12])

== system cpp_m1hp_demo/M1 CPP/HP selector ==
  In1 : Inport
  Selector : Selector  InputPortWidth=12  IndexOptions=Index vector (dialog)  Indices=[1:6:12]  OutputSizes=1
  Selector1 : Selector  InputPortWidth=12  IndexOptions=Index vector (dialog)  Indices=[2:6:12]  OutputSizes=1
  Selector2 : Selector  InputPortWidth=12  IndexOptions=Index vector (dialog)  Indices=[3:6:12]  OutputSizes=1
  Selector3 : Selector  InputPortWidth=12  IndexOptions=Index vector (dialog)  Indices=[4:6:12]  OutputSizes=1
  Selector4 : Selector  InputPortWidth=12  IndexOptions=Index vector (dialog)  Indices=[5:6:12]  OutputSizes=1
  Selector5 : Selector  InputPortWidth=12  IndexOptions=Index vector (dialog)  Indices=[6:6:12]  OutputSizes=1
  HP1 : Outport  VectorParamsAs1DForOutWhenUnconnected=off
  HP2 : Outport  Port=2  VectorParamsAs1DForOutWhenUnconnected=off
  HP3 : Outport  Port=3  VectorParamsAs1DForOutWhenUnconnected=off
  HP4 : Outport  Port=4  VectorParamsAs1DForOutWhenUnconnected=off
  HP5 : Outport  Port=5  VectorParamsAs1DForOutWhenUnconnected=off
  HP6 : Outport  Port=6  VectorParamsAs1DForOutWhenUnconnected=off
  wires:
  In1/1 -> Selector3/1, Selector2/1, Selector4/1, Selector5/1, Selector/1, Selector1/1
  Selector/1 -> HP1/1
  Selector5/1 -> HP6/1
  Selector1/1 -> HP2/1
  Selector2/1 -> HP3/1
  Selector3/1 -> HP4/1
  Selector4/1 -> HP5/1

== system cpp_m1hp_demo/M1 CPP/cmd_pre_proc ==
  x_target : Inport
  v_target : Inport  Port=2
  Bessel filter : Subsystem  TreatAsAtomicUnit=on
  CPP with multi-axis coordination : Subsystem  TreatAsAtomicUnit=on
  CPP with multi-axis coordination1 : Subsystem  TreatAsAtomicUnit=on
  Compare To Zero : simulink/Logic and Bit Operations/Compare To Zero  relop===  OutDataTypeStr=boolean
  Motion equations : Subsystem  TreatAsAtomicUnit=on
  Sample_generator : Subsystem
  Scope : Scope  NumInputPorts=3
  Scope1 : Scope  NumInputPorts=3
  Triggered Subsystem : Subsystem  TreatAsAtomicUnit=on
  pos_d : Outport  VectorParamsAs1DForOutWhenUnconnected=off
  vel_d : Outport  Port=2  VectorParamsAs1DForOutWhenUnconnected=off
  acc_d : Outport  Port=3  VectorParamsAs1DForOutWhenUnconnected=off
  wires:
  x_target/1 -> Triggered Subsystem/1(x1_multi_ax)
  v_target/1 -> Triggered Subsystem/4(v1_multi_ax)
  Triggered Subsystem/1(k_a_ac_acd) -> CPP with multi-axis coordination1/2(k_acd), CPP with multi-axis coordination/2(k_acd)
  Triggered Subsystem/2(max_bool) -> CPP with multi-axis coordination/3(max_bool)
  Triggered Subsystem/3(a_l) -> CPP with multi-axis coordination/4(acc_l)
  Triggered Subsystem/4(Dx) -> CPP with multi-axis coordination/5(Dx)
  Triggered Subsystem/5(Dv) -> CPP with multi-axis coordination/6(Dv)
  Compare To Zero/1 -> Scope1/2, Triggered Subsystem/Trigger
  Motion equations/2(vel_d_vec) -> Triggered Subsystem/3(v0_multi_ax), Scope/2, Bessel filter/2(vel_vec)
  Bessel filter/1(pos_f_vec) -> pos_d/1
  Bessel filter/2(vel_f_vec) -> vel_d/1
  Bessel filter/3(acc_f_vec) -> acc_d/1
  CPP with multi-axis coordination/1(multi_ax_acc_d) -> Scope1/3, Motion equations/1(acc_d), Scope/1, Bessel filter/3(acc_vec)
  Sample_generator/1(k) -> Compare To Zero/1, CPP with multi-axis coordination1/1(k), CPP with multi-axis coordination/1(k), Scope1/1, Motion equations/2(k)
  CPP with multi-axis coordination1/1(Dk) -> Motion equations/3(Dk)
  Motion equations/1(pos_d_vec) -> Triggered Subsystem/2(x0_multi_ax), Scope/3, Bessel filter/1(pos_vec)

== system cpp_m1hp_demo/M1_HP_loadcells/M1S1 Loadcell ==
  note: HP Forces
  note: HP Relative
      | Displacements
  HP_F_cmd : Inport
  HP_D_cell : Inport  Port=2
  HP_D_face : Inport  Port=3
  HpK : Gain  Gain=m1sys{1}.HPstiff
  Sum1 : Sum  Inputs=-+|
  Sum9 : Sum  Inputs=-+|
  HP_F_meas : Outport  VectorParamsAs1DForOutWhenUnconnected=off
  wires:
  HP_D_cell/1 -> Sum9/1
  HP_D_face/1 -> Sum9/2
  Sum9/1 -> HpK/1
  HpK/1 -> Sum1/2
  Sum1/1 -> HP_F_meas/1
  HP_F_cmd/1 -> Sum1/1

== system cpp_m1hp_demo/M1_HP_loadcells/M1S2 Loadcell ==
  note: HP Relative
      | Displacements
  note: HP Forces
  HP_F_cmd : Inport
  HP_D_cell : Inport  Port=2
  HP_D_face : Inport  Port=3
  HpK : Gain  Gain=m1sys{2}.HPstiff
  Sum1 : Sum  Inputs=-+|
  Sum9 : Sum  Inputs=-+|
  HP_F_meas : Outport  VectorParamsAs1DForOutWhenUnconnected=off
  wires:
  HP_D_face/1 -> Sum9/2
  HP_D_cell/1 -> Sum9/1
  HP_F_cmd/1 -> Sum1/1
  HpK/1 -> Sum1/2
  Sum1/1 -> HP_F_meas/1
  Sum9/1 -> HpK/1

== system cpp_m1hp_demo/M1_HP_loadcells/M1S3 Loadcell ==
  note: HP Relative
      | Displacements
  note: HP Forces
  HP_F_cmd : Inport
  HP_D_cell : Inport  Port=2
  HP_D_face : Inport  Port=3
  HpK : Gain  Gain=m1sys{3}.HPstiff
  Sum1 : Sum  Inputs=-+|
  Sum9 : Sum  Inputs=-+|
  HP_F_meas : Outport  VectorParamsAs1DForOutWhenUnconnected=off
  wires:
  HP_D_face/1 -> Sum9/2
  HP_D_cell/1 -> Sum9/1
  HP_F_cmd/1 -> Sum1/1
  HpK/1 -> Sum1/2
  Sum1/1 -> HP_F_meas/1
  Sum9/1 -> HpK/1

== system cpp_m1hp_demo/M1_HP_loadcells/M1S4 Loadcell ==
  note: HP Relative
      | Displacements
  note: HP Forces
  HP_F_cmd : Inport
  HP_D_cell : Inport  Port=2
  HP_D_face : Inport  Port=3
  HpK : Gain  Gain=m1sys{4}.HPstiff
  Sum1 : Sum  Inputs=-+|
  Sum9 : Sum  Inputs=-+|
  HP_F_meas : Outport  VectorParamsAs1DForOutWhenUnconnected=off
  wires:
  HP_D_face/1 -> Sum9/2
  HP_D_cell/1 -> Sum9/1
  HP_F_cmd/1 -> Sum1/1
  HpK/1 -> Sum1/2
  Sum1/1 -> HP_F_meas/1
  Sum9/1 -> HpK/1

== system cpp_m1hp_demo/M1_HP_loadcells/M1S5 Loadcell ==
  note: HP Relative
      | Displacements
  note: HP Forces
  HP_F_cmd : Inport
  HP_D_cell : Inport  Port=2
  HP_D_face : Inport  Port=3
  HpK : Gain  Gain=m1sys{5}.HPstiff
  Sum1 : Sum  Inputs=-+|
  Sum9 : Sum  Inputs=-+|
  HP_F_meas : Outport  VectorParamsAs1DForOutWhenUnconnected=off
  wires:
  HP_D_face/1 -> Sum9/2
  HP_D_cell/1 -> Sum9/1
  HP_F_cmd/1 -> Sum1/1
  HpK/1 -> Sum1/2
  Sum1/1 -> HP_F_meas/1
  Sum9/1 -> HpK/1

== system cpp_m1hp_demo/M1_HP_loadcells/M1S6 Loadcell ==
  note: HP Relative
      | Displacements
  note: HP Forces
  HP_F_cmd : Inport
  HP_D_cell : Inport  Port=2
  HP_D_face : Inport  Port=3
  HpK : Gain  Gain=m1sys{6}.HPstiff
  Sum1 : Sum  Inputs=-+|
  Sum9 : Sum  Inputs=-+|
  HP_F_meas : Outport  VectorParamsAs1DForOutWhenUnconnected=off
  wires:
  HP_D_face/1 -> Sum9/2
  HP_D_cell/1 -> Sum9/1
  HP_F_cmd/1 -> Sum1/1
  HpK/1 -> Sum1/2
  Sum1/1 -> HP_F_meas/1
  Sum9/1 -> HpK/1

== system cpp_m1hp_demo/M1_HP_loadcells/M1S7 Control ==
  note: HP Relative
      | Displacements
  note: HP Forces
  HP_F_cmd : Inport
  HP_D_cell : Inport  Port=2
  HP_D_face : Inport  Port=3
  HpK : Gain  Gain=m1sys{7}.HPstiff
  Sum1 : Sum  Inputs=-+|
  Sum9 : Sum  Inputs=-+|
  HP_F_meas : Outport  VectorParamsAs1DForOutWhenUnconnected=off
  wires:
  HP_D_face/1 -> Sum9/2
  HP_D_cell/1 -> Sum9/1
  HP_F_cmd/1 -> Sum1/1
  HpK/1 -> Sum1/2
  Sum1/1 -> HP_F_meas/1
  Sum9/1 -> HpK/1

== system cpp_m1hp_demo/Mount_Control/DT_siso_SS ==
  In1 : Inport
  A : Gain  Gain=a  Multiplication=Matrix(K*u) (u vector)
  Add : Sum
  B : Gain  Gain=b
  C : Gain  Gain=c
  Unit Delay : UnitDelay  SampleTime=-1  HasFrameUpgradeWarning=on
  Out1 : Outport
  wires:
  In1/1 -> B/1
  C/1 -> Out1/1
  B/1 -> Add/1
  Add/1 -> Unit Delay/1
  A/1 -> Add/2
  Unit Delay/1 -> A/1, C/1

== system cpp_m1hp_demo/Mount_Drv_FDR2023_linear/DRV Friction ==
  AxisVel_rad/s : Inport
  AZ DT Lugre Fr mode : Subsystem  mask{sigma0=az.oFr.sigm0, sigma1=az.oFr.sigm1, Tc=az.oFr.Tc, sigmav=az.oFr.sigmv, Ts=az.oFr.Ts, vs=az.oFr.vs, iIsSig01Active=az.oFr.iIsSig01Active}
      mask prompts: iIsSig01Active "0=inactive, 1=active"
  Constant : Constant  Value=o.az.oFr.bIsActive
  Constant1 : Constant  Value=o.el.oFr.bIsActive
  Constant3 : Constant  Value=o.gir.oFr.bIsActive
  Demux5 : Demux  Outputs=[1,1,1]
  EL DT Lugre Fr model : Subsystem  mask{sigma0=el.oFr.sigm0, sigma1=el.oFr.sigm1, Tc=el.oFr.Tc, sigmav=el.oFr.sigmv, Ts=el.oFr.Ts, vs=el.oFr.vs, iIsSig01Active=el.oFr.iIsSig01Active}
      mask prompts: iIsSig01Active "0=inactive, 1=active"
  EL DT Lugre Fr model_ : Subsystem  Commented=on  TreatAsAtomicUnit=on  mask{frParStruct=mount.el.Fr}
      mask prompts: frParStruct "Structure with the Friction model parameters"
  GIR DT Lugre Fr model : Subsystem  mask{sigma0=gir.oFr.sigm0, sigma1=gir.oFr.sigm1, Tc=gir.oFr.Tc, sigmav=gir.oFr.sigmv, Ts=gir.oFr.Ts, vs=gir.oFr.vs, iIsSig01Active=gir.oFr.iIsSig01Active}
      mask prompts: iIsSig01Active "0=inactive, 1=active"
  GIR DT Lugre Fr model_ : Subsystem  Commented=on  TreatAsAtomicUnit=on  mask{frParStruct=mount.gir.Fr}
      mask prompts: frParStruct "Structure with the Friction model parameters"
  Mux1 : Mux  Inputs=[1,1,1]
  Friction_To : Outport
  wires:
  Demux5/3 -> GIR DT Lugre Fr model/1(v)
  Demux5/2 -> EL DT Lugre Fr model/1(v)
  Demux5/1 -> AZ DT Lugre Fr mode/1(v)
  AxisVel_rad/s/1 -> Demux5/1
  Constant1/1 -> EL DT Lugre Fr model/Enable
  GIR DT Lugre Fr model/1(Tfr) -> Mux1/3
  AZ DT Lugre Fr mode/1(Tfr) -> Mux1/1
  Constant3/1 -> GIR DT Lugre Fr model/Enable
  Constant/1 -> AZ DT Lugre Fr mode/Enable
  EL DT Lugre Fr model/1(Tfr) -> Mux1/2
  Mux1/1 -> Friction_To/1

== system cpp_m1hp_demo/Mount_Drv_FDR2023_linear/Friction ==
  Vel : Inport
  Enable : EnablePort
  Constant : Constant  Value=az.oFr.bIsActive
  Constant1 : Constant  Value=el.oFr.bIsActive
  Constant2 : Constant  Value=gir.oFr.bIsActive
  Demux1 : Demux  Outputs=3
  Friction Alt : Subsystem  mask{sigma0=el.oFr.sigm0, sigma1=el.oFr.sigm1, Tc=el.oFr.Tc, sigmav=el.oFr.sigmv, Ts=el.oFr.Ts, vs=el.oFr.vs, iIsSig01Active=el.oFr.iIsSig01Active}
      mask prompts: iIsSig01Active "0=inactive, 1=active"
  Friction Az : Subsystem  mask{sigma0=az.oFr.sigm0, sigma1=az.oFr.sigm1, Tc=az.oFr.Tc, sigmav=az.oFr.sigmv, Ts=az.oFr.Ts, vs=az.oFr.vs, iIsSig01Active=az.oFr.iIsSig01Active}
      mask prompts: iIsSig01Active "0=inactive, 1=active"
  Friction Gir : Subsystem  mask{sigma0=gir.oFr.sigm0, sigma1=gir.oFr.sigm1, Tc=gir.oFr.Tc, sigmav=gir.oFr.sigmv, Ts=gir.oFr.Ts, vs=gir.oFr.vs, iIsSig01Active=gir.oFr.iIsSig01Active}
      mask prompts: iIsSig01Active "0=inactive, 1=active"
  Mux2 : Mux  Inputs=3
  Unit Delay : UnitDelay  SampleTime=-1  HasFrameUpgradeWarning=on
  FrictionTo : Outport
  wires:
  Friction Alt/1(Tfr) -> Mux2/2
  Demux1/2 -> Friction Alt/1(v)
  Demux1/1 -> Friction Az/1(v)
  Friction Az/1(Tfr) -> Mux2/1
  Mux2/1 -> FrictionTo/1
  Constant1/1 -> Friction Alt/Enable
  Constant/1 -> Friction Az/Enable
  Constant2/1 -> Friction Gir/Enable
  Demux1/3 -> Friction Gir/1(v)
  Unit Delay/1 -> Demux1/1
  Vel/1 -> Unit Delay/1
  Friction Gir/1(Tfr) -> Mux2/3

== system cpp_m1hp_demo/Mount_Drv_FDR2023_linear/Parasitic torque model ==
  Axis_Pos_rad : Inport
  Drv_To : Inport  Port=2
  Constant1 : Constant  Value=az.oParasitic.bIsActive
  Constant2 : Constant  Value=el.oParasitic.bIsActive
  Constant3 : Constant  Value=gir.oParasitic.bIsActive
  Demux : Demux  Outputs=[1,1,1]
  Demux1 : Demux  Outputs=[1,1,1]
  Mux3 : Mux  Inputs=3
  Parasitic AZ : Subsystem  mask{oParasitic=az.oParasitic}
  Parasitic EL : Subsystem  mask{oParasitic=el.oParasitic}
  Parasitic GIR : Subsystem  mask{oParasitic=gir.oParasitic}
  Radians to Degrees : simulink_extras/Transformations/Radians to Degrees
  UnitDelay_PO : UnitDelay  Commented=through  SampleTime=-1  HasFrameUpgradeWarning=on
  UnitDelay_To : UnitDelay  Commented=through  SampleTime=-1  HasFrameUpgradeWarning=on
  ParasiticTo : Outport
  wires:
  Demux/1 -> Parasitic AZ/2(AxisPo_deg)
  Demux/2 -> Parasitic EL/2(AxisPo_deg)
  Demux/3 -> Parasitic GIR/2(AxisPo_deg)
  UnitDelay_PO/1 -> Radians to Degrees/1
  UnitDelay_To/1 -> Demux1/1
  Demux1/3 -> Parasitic GIR/1(AxisTo_Nm)
  Demux1/2 -> Parasitic EL/1(AxisTo_Nm)
  Demux1/1 -> Parasitic AZ/1(AxisTo_Nm)
  Drv_To/1 -> UnitDelay_To/1
  Constant2/1 -> Parasitic EL/Enable
  Parasitic EL/1(TotalTo) -> Mux3/2
  Radians to Degrees/1 -> Demux/1
  Constant3/1 -> Parasitic GIR/Enable
  Axis_Pos_rad/1 -> UnitDelay_PO/1
  Parasitic GIR/1(TotalTo) -> Mux3/3
  Constant1/1 -> Parasitic AZ/Enable
  Parasitic AZ/1(TotalTo) -> Mux3/1
  Mux3/1 -> ParasiticTo/1

== system cpp_m1hp_demo/Mount_Drv_FDR2023_linear/ToothContact Torques ==
  AxisPo_rad : Inport
  AxisTo : Inport  Port=2
  Constant2 : Constant  Value=[0 0]
  Mux3 : Mux  Inputs=2
  Radians to Degrees : simulink_extras/Transformations/Radians to Degrees
  Sel : Selector  InputPortWidth=3  IndexOptions=Index vector (dialog)  Indices=[3]  OutputSizes=1
  Sel1 : Selector  InputPortWidth=3  IndexOptions=Index vector (dialog)  Indices=[3]  OutputSizes=1
  Sum1 : Sum  Inputs=|++
  ToothContact GIR (Norm) : Subsystem  mask{oToothContact=gir.oToothContactNorm}
  ToothContact GIR (Peak) : Subsystem  mask{oToothContact=gir.oToothContactPeak}
  factAxial : Gain  Gain=gir.oToothContactPeak.factAxial
  ToothContactTo : Outport
  ToothContactAxialFo : Outport  Port=2
  wires:
  ToothContact GIR (Norm)/1(TotalTo) -> Sum1/2
  Sum1/1 -> Mux3/2, factAxial/1
  Sel/1 -> Radians to Degrees/1
  Radians to Degrees/1 -> ToothContact GIR (Peak)/1(AxisPos_deg), ToothContact GIR (Norm)/1(AxisPos_deg)
  Sel1/1 -> ToothContact GIR (Peak)/2(AxisTo), ToothContact GIR (Norm)/2(AxisTo)
  Mux3/1 -> ToothContactTo/1
  AxisTo/1 -> Sel1/1
  AxisPo_rad/1 -> Sel/1
  factAxial/1 -> ToothContactAxialFo/1
  ToothContact GIR (Peak)/1(TotalTo) -> Sum1/1
  Constant2/1 -> Mux3/1

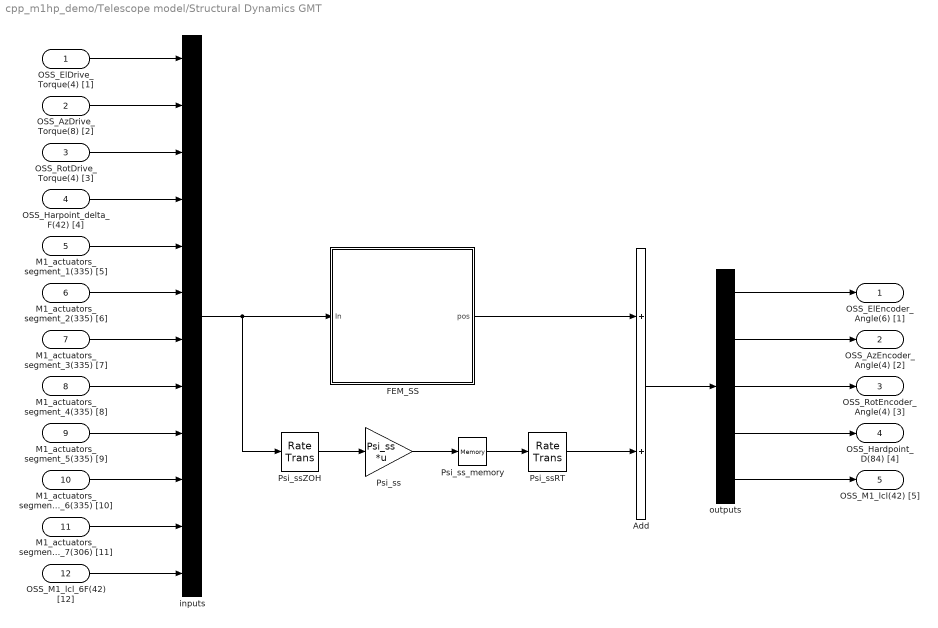
== system cpp_m1hp_demo/Telescope model/Structural Dynamics GMT ==
  OSS_ElDrive_Torque(4) [1] : Inport  PortDimensions=4
  OSS_AzDrive_Torque(8) [2] : Inport  Port=2  PortDimensions=8
  OSS_RotDrive_Torque(4) [3] : Inport  Port=3  PortDimensions=4
  OSS_Harpoint_delta_F(42) [4] : Inport  Port=4  PortDimensions=42
  M1_actuators_segment_1(335) [5] : Inport  Port=5  PortDimensions=335
  M1_actuators_segment_2(335) [6] : Inport  Port=6  PortDimensions=335
  M1_actuators_segment_3(335) [7] : Inport  Port=7  PortDimensions=335
  M1_actuators_segment_4(335) [8] : Inport  Port=8  PortDimensions=335
  M1_actuators_segment_5(335) [9] : Inport  Port=9  PortDimensions=335
  M1_actuators_segment_6(335) [10] : Inport  Port=10  PortDimensions=335
  M1_actuators_segment_7(306) [11] : Inport  Port=11  PortDimensions=306
  OSS_M1_lcl_6F(42) [12] : Inport  Port=12  PortDimensions=42
  Add : Sum
  FEM_SS : Subsystem
  Psi_ss : Gain  Gain=Psi_ss  Multiplication=Matrix(K*u) (u vector)
  Psi_ssRT : RateTransition  Integrity=off  OutPortSampleTimeOpt=Inherit
  Psi_ssZOH : RateTransition  Integrity=off  OutPortSampleTime=Psi_ssTs
  Psi_ss_memory : Memory  InitialCondition=zeros(size(phiC,1),1)  InheritSampleTime=on  LinearizeAsDelay=on
  inputs : Mux  Inputs=modelMuxDims
  outputs : Demux  Outputs=modelDemuxDims
  OSS_ElEncoder_Angle(6) [1] : Outport  PortDimensions=6
  OSS_AzEncoder_Angle(4) [2] : Outport  Port=2  PortDimensions=4
  OSS_RotEncoder_Angle(4) [3] : Outport  Port=3  PortDimensions=4
  OSS_Hardpoint_D(84) [4] : Outport  Port=4  PortDimensions=84
  OSS_M1_lcl(42) [5] : Outport  Port=5  PortDimensions=42
  wires:
  outputs/5 -> OSS_M1_lcl(42) [5]/1
  outputs/4 -> OSS_Hardpoint_D(84) [4]/1
  outputs/3 -> OSS_RotEncoder_Angle(4) [3]/1
  outputs/2 -> OSS_AzEncoder_Angle(4) [2]/1
  outputs/1 -> OSS_ElEncoder_Angle(6) [1]/1
  OSS_M1_lcl_6F(42) [12]/1 -> inputs/12
  M1_actuators_segment_7(306) [11]/1 -> inputs/11
  M1_actuators_segment_6(335) [10]/1 -> inputs/10
  M1_actuators_segment_5(335) [9]/1 -> inputs/9
  M1_actuators_segment_4(335) [8]/1 -> inputs/8
  M1_actuators_segment_3(335) [7]/1 -> inputs/7
  M1_actuators_segment_2(335) [6]/1 -> inputs/6
  M1_actuators_segment_1(335) [5]/1 -> inputs/5
  OSS_Harpoint_delta_F(42) [4]/1 -> inputs/4
  OSS_RotDrive_Torque(4) [3]/1 -> inputs/3
  OSS_AzDrive_Torque(8) [2]/1 -> inputs/2
  OSS_ElDrive_Torque(4) [1]/1 -> inputs/1
  Psi_ss/1 -> Psi_ss_memory/1
  FEM_SS/1(pos) -> Add/1
  Add/1 -> outputs/1
  Psi_ssZOH/1 -> Psi_ss/1
  Psi_ss_memory/1 -> Psi_ssRT/1
  Psi_ssRT/1 -> Add/2
  inputs/1 -> Psi_ssZOH/1, FEM_SS/1(In)

== system cpp_m1hp_demo/M1 CPP/cmd_pre_proc/Bessel filter ==
  pos_vec : Inport  Partition=on  PartitionDimension=1  PartitionWidth=1  PartitionOffset=0
  vel_vec : Inport  Port=2  Partition=on  PartitionDimension=1  PartitionWidth=1  PartitionOffset=0
  acc_vec : Inport  Port=3  Partition=on  PartitionDimension=1  PartitionWidth=1  PartitionOffset=0
  For Each : ForEach  DisableCoverage=on  SpecifiedNumIters=n_in
  Jerk-limitation : Subsystem
  pos_f_vec : Outport  ConcatenationDimension=1
  vel_f_vec : Outport  Port=2  ConcatenationDimension=1
  acc_f_vec : Outport  Port=3  ConcatenationDimension=1
  wires:
  vel_vec/1 -> Jerk-limitation/2(vel)
  Jerk-limitation/3(pos_f) -> pos_f_vec/1
  Jerk-limitation/2(vel_f) -> vel_f_vec/1
  Jerk-limitation/1(acc_f) -> acc_f_vec/1
  pos_vec/1 -> Jerk-limitation/3(pos)
  acc_vec/1 -> Jerk-limitation/1(acc)

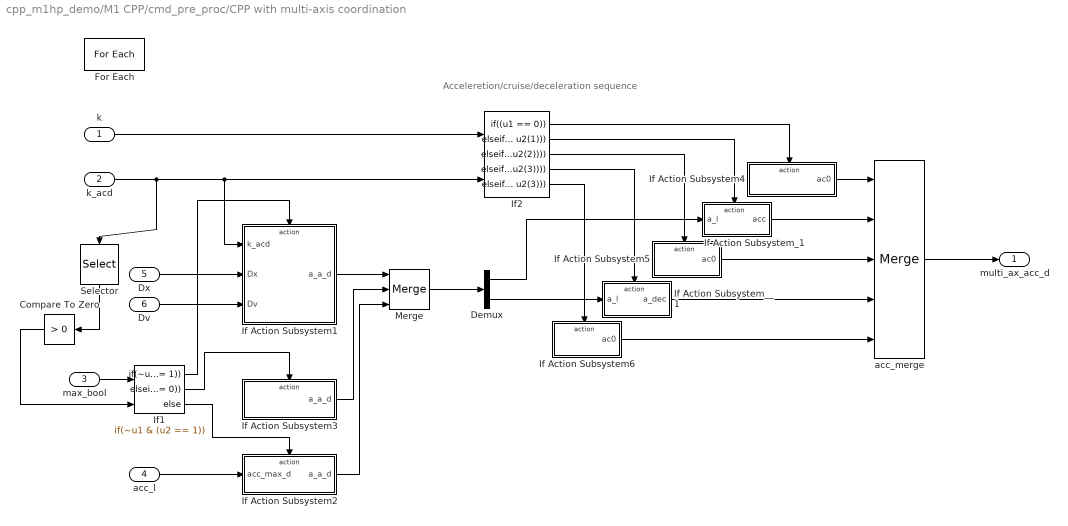
== system cpp_m1hp_demo/M1 CPP/cmd_pre_proc/CPP with multi-axis coordination ==
  note: Acceleretion/cruise/deceleration sequence
  k : Inport
  k_acd : Inport  Port=2
  max_bool : Inport  Port=3  Partition=on  PartitionDimension=1  PartitionWidth=1  PartitionOffset=0
  acc_l : Inport  Port=4  Partition=on  PartitionDimension=1  PartitionWidth=1  PartitionOffset=0
  Dx : Inport  Port=5  Partition=on  PartitionDimension=1  PartitionWidth=1  PartitionOffset=0
  Dv : Inport  Port=6  Partition=on  PartitionDimension=1  PartitionWidth=1  PartitionOffset=0
  Compare To Zero : simulink/Logic and Bit Operations/Compare To Zero  relop=>  OutDataTypeStr=boolean
  Demux : Demux  Outputs=2
  For Each : ForEach  DisableCoverage=on
  If Action Subsystem1 : Subsystem  TreatAsAtomicUnit=on
  If Action Subsystem2 : Subsystem  TreatAsAtomicUnit=on
  If Action Subsystem3 : Subsystem  TreatAsAtomicUnit=on
  If Action Subsystem4 : Subsystem  TreatAsAtomicUnit=on
  If Action Subsystem5 : Subsystem  TreatAsAtomicUnit=on
  If Action Subsystem6 : Subsystem  TreatAsAtomicUnit=on
  If Action Subsystem_1 : Subsystem  TreatAsAtomicUnit=on
  If Action Subsystem__1 : Subsystem  TreatAsAtomicUnit=on
  If1 : If  NumInputs=2  IfExpression=~u1 & (u2 == 1)  ElseIfExpressions=~u1 & (u2 == 0)
  If2 : If  NumInputs=2  IfExpression=(u1 == 0)  ElseIfExpressions=(u1 <= u2(1)), ((u1 > u2(1)) & (u1 <= u2(2))), ((u1 > u2(2)) & (u1 <= u2(3))), (u1 > u2(3))  ShowElse=off
  Merge : Merge  Inputs=3
  Selector : Selector  InputPortWidth=3  IndexOptions=Index vector (dialog)  Indices=[3]  OutputSizes=1
  acc_merge : Merge  Inputs=5  InitialOutput=0
  multi_ax_acc_d : Outport  ConcatenationDimension=1
  wires:
  acc_merge/1 -> multi_ax_acc_d/1
  k/1 -> If2/1
  max_bool/1 -> If1/1
  If1/1 -> If Action Subsystem1/Action
  If1/3 -> If Action Subsystem2/Action
  acc_l/1 -> If Action Subsystem2/1(acc_max_d)
  If Action Subsystem2/1(a_a_d) -> Merge/3
  If Action Subsystem1/1(a_a_d) -> Merge/1
  Merge/1 -> Demux/1
  Dx/1 -> If Action Subsystem1/2(Dx)
  Dv/1 -> If Action Subsystem1/3(Dv)
  If Action Subsystem3/1(a_a_d) -> Merge/2
  Selector/1 -> Compare To Zero/1
  If1/2 -> If Action Subsystem3/Action
  Compare To Zero/1 -> If1/2
  If Action Subsystem5/1(ac0) -> acc_merge/3
  If2/1 -> If Action Subsystem4/Action
  Demux/2 -> If Action Subsystem__1/1(a_l)
  If Action Subsystem4/1(ac0) -> acc_merge/1
  If2/3 -> If Action Subsystem5/Action
  If2/4 -> If Action Subsystem__1/Action
  If Action Subsystem__1/1(a_dec) -> acc_merge/4
  If2/2 -> If Action Subsystem_1/Action
  If Action Subsystem_1/1(acc) -> acc_merge/2
  Demux/1 -> If Action Subsystem_1/1(a_l)
  If2/5 -> If Action Subsystem6/Action
  If Action Subsystem6/1(ac0) -> acc_merge/5
  k_acd/1 -> If2/2, If Action Subsystem1/1(k_acd), Selector/1
